simulink model "Simscape_crane_software_model_RealSensors_R2016a"  (R2016a)
settings: Solver=ode15s  StartTime=0.0  StopTime=120  RelTol=1e-3
values from neighbouring files (symbols this model uses):
  DOsc = 0.01    [RunModel.m]    (also in RunModelVerification.m)
  DTraj = 0.3    [RunModel.m]    (also in RunModelVerification.m)
  IOsc = 0    [RunModel.m]    (also in RunModelVerification.m)
  ITraj = 0.3    [RunModel.m]    (also in RunModelVerification.m)
  POsc = 0.9    [RunModel.m]    (also in RunModelVerification.m)
  PTraj = 3.0    (= 3)    [RunModel.m]    (also in RunModelVerification.m)
  waypoints = [waypoints, find_nearest_obstacles(waypoints, Grid)]    [path_planning.m]    (also in path_to_waypoints.m = [])
undefined symbols (not defined in the file or in its folder): m, MR, TxBreak, TxCoulomb, TxVisc, TyBreak, TyCoulomb, TzBreak, TzCoulomb, X, xRange, xZero, Y, yRange, yZero, Z, zRange, zZero
undefined symbols (not defined in the file): M, TorqueMultX, TorqueMultY, TorqueMultZ, TxTrans, TyTrans, TyVisc, TzTrans, TzVisc
libraries: sm_lib x146, fl_lib x62, nesl_utility x24, simulink x10, elec_lib x9, sm_double_wishbone_suspension_lib x4, aerolibtransform2 x1
(part 1 of 14)
settings Model: Creator=jsustare  LastModifiedBy=Jukka
settings SolverCC: MaxConsecutiveMinStep=10
settings DataIOCC: SaveFormat=StructureWithTime
settings DebuggingCC: AllowSymbolicDim=off
settings ModelReferenceCC: PropagateSignalLabelsOutOfModel=off
settings GRTTargetCC: GeneratePreprocessorConditionals=Use local settings
settings SimscapeCC: SimscapeLogType=all
settings ConfigurationSet: Description=SimMechanics 2G
settings ExplorerConfigSet: SimMechanicsOpenEditorOnUpdate=off

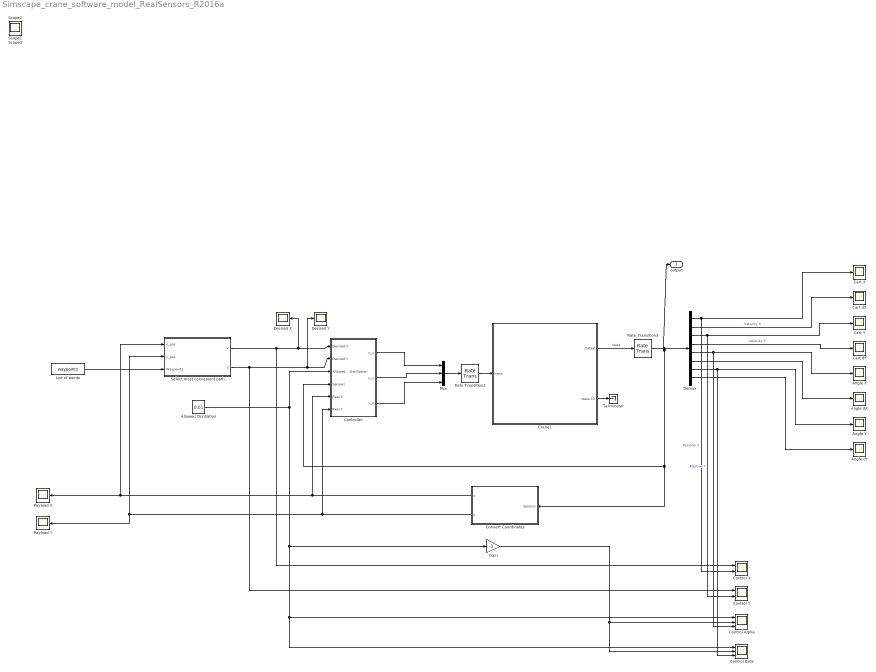
== system Simscape_crane_software_model_RealSensors_R2016a ==
  Allowed Oscillation : Constant  Value=0.01
  Angle X : Scope
  Angle Y : Scope
  Angle dX : Scope
  Angle dY : Scope
  Cart X : Scope
  Cart Y : Scope
  Cart dX : Scope
  Cart dY : Scope
  Control Alpha : Scope  NumInputPorts=3
  Control Beta : Scope  NumInputPorts=3
  Control X : Scope  NumInputPorts=2
  Control Y : Scope  NumInputPorts=2
  Controller : Subsystem
  Convert Coordinates : MATLAB Function  TreatAsAtomicUnit=on
  Crane1 : Subsystem  mask{penduMass=m, cartMass=M, MR=MR, xRange=xRange, yRange=yRange, zRange=zRange, xZero=xZero, yZero=yZero, zZero=zZero, TxBreak=TxBreak, TxCoulomb=TxCoulomb, TxVisc=TxVisc, TxTrans=TxTrans, TyBreak=TyBreak, TyCoulomb=TyCoulomb, TyVisc=TyVisc, TyTrans=TyTrans, TzBreak=TzBreak, TzCoulomb=TzCoulomb, TzVisc=TzVisc, TzTrans=TzTrans, Ux=TorqueMultX, Uy=TorqueMultY, Uz=TorqueMultZ}
      mask prompts: penduMass "Pendulum Mass (Kg)"; cartMass "Mass of the cart (Kg)"; MR "Mass of the rail (Kg)"; TxBreak "BreakAwayFriction"; TxCoulomb "Coulomb Friction"; TxVisc "Viscous friction"; TxTrans "Transition coeff"; TyBreak "BreakAwayFriction"; TyCoulomb "Coulomb Friction"; TyVisc "Viscous friction"; TyTrans "Transition coeff"; TzBreak "BreakAwayFriction"; TzCoulomb "Coulomb Friction"; TzVisc "Viscous friction"; TzTrans "Transition coeff"; Ux "Rail motor multiplier (X)"; Uy "Cart motor multiplier (Y)"; Uz "String motor multiplier (Z)"
      mask init:
      | %mass lowSat
      | penduMass=max(penduMass,1e-3);
      | cartMass=max(cartMass,1e-3);
      | MR=max(MR,1e-3);
      | 
      | %zeros saturated
      | xZero=max(xZero,xRange(1));
      | xZero=min(xZero,xRange(2));
      | 
      | yZero=max(yZero,yRange(1));
      | yZero=min(yZero,yRange(2));
      | 
      | zZero=max(zZero,zRange(1));
      | zZero=min(zZero,zRange(2));
      mask DialogControl DescGroupVar Prompt: 3D Crane Simscape model
      mask Display:
